simulink model "S2"  (R2021b)
settings: Solver=VariableStepAuto  StartTime=0.0  StopTime=6  RelTol=1e-3
settings Model: Creator=m433  LastModifiedBy=hp
settings SolverCC: AlgebraicLoopSolver=TrustRegion
settings DebuggingCC: SFMachineParentedDataDiag=warning

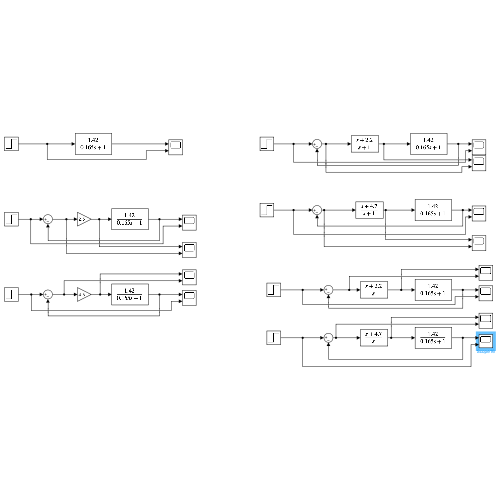
[thumbnail: Simulink's stored preview of the top-level diagram]
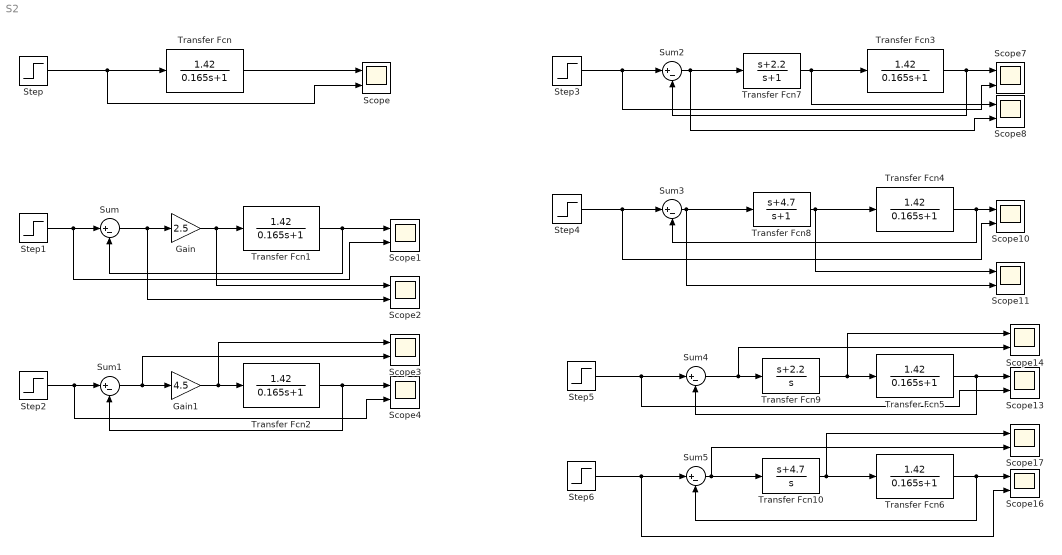
== system S2 ==
  Gain : Gain  Gain=2.5
  Gain1 : Gain  Gain=4.5
  Scope{,1..4,7..8,10..11,13..14,16..17} (13 alike) : Scope  NumInputPorts=2
  Step : Step  Time=0  After=4  SampleTime=0
  Step1 : Step  Time=0.5  Before=-4  After=4  SampleTime=0
  Step2 : Step  Time=0.5  Before=-4  After=4  SampleTime=0
  Step3 : Step  Time=3.5  Before=-4  After=4  SampleTime=0
  Step4 : Step  Time=1.5  Before=-4  After=4  SampleTime=0
  Step5 : Step  Time=5  Before=-4  After=4  SampleTime=0
  Step6 : Step  Time=3  Before=-4  After=4  SampleTime=0
  Sum{,1..5} (6 alike) : Sum  Inputs=|+-
  Transfer Fcn{,1..6} (7 alike) : TransferFcn  Numerator=[1.42]  Denominator=[0.165 1]
  Transfer Fcn10 : TransferFcn  Numerator=[1 4.7]  Denominator=[1 0]
  Transfer Fcn7 : TransferFcn  Numerator=[1 2.2]  Denominator=[1 1]
  Transfer Fcn8 : TransferFcn  Numerator=[1 4.7]  Denominator=[1 1]
  Transfer Fcn9 : TransferFcn  Numerator=[1 2.2]  Denominator=[1 0]
  wires:
  Sum2/1 -> Scope8/2, Transfer Fcn7/1
  Transfer Fcn7/1 -> Scope8/1, Transfer Fcn3/1
  Sum/1 -> Scope2/2, Gain/1
  Gain/1 -> Scope2/1, Transfer Fcn1/1
  Sum1/1 -> Scope3/2, Gain1/1
  Gain1/1 -> Scope3/1, Transfer Fcn2/1
  Transfer Fcn2/1 -> Scope4/1, Sum1/2
  Step1/1 -> Scope1/2, Sum/1
  Transfer Fcn1/1 -> Scope1/1, Sum/2
  Transfer Fcn3/1 -> Scope7/1, Sum2/2
  Transfer Fcn8/1 -> Scope11/1, Transfer Fcn4/1
  Sum3/1 -> Scope11/2, Transfer Fcn8/1
  Transfer Fcn4/1 -> Scope10/1, Sum3/2
  Sum4/1 -> Scope14/2, Transfer Fcn9/1
  Transfer Fcn9/1 -> Scope14/1, Transfer Fcn5/1
  Transfer Fcn5/1 -> Scope13/1, Sum4/2
  Sum5/1 -> Scope17/2, Transfer Fcn10/1
  Transfer Fcn10/1 -> Scope17/1, Transfer Fcn6/1
  Transfer Fcn6/1 -> Scope16/1, Sum5/2
  Transfer Fcn/1 -> Scope/1
  Step/1 -> Transfer Fcn/1, Scope/2
  Step2/1 -> Sum1/1, Scope4/2
  Step3/1 -> Sum2/1, Scope7/2
  Step4/1 -> Sum3/1, Scope10/2
  Step5/1 -> Sum4/1, Scope13/2
  Step6/1 -> Sum5/1, Scope16/2
